simulink model "AQLRL"  (R2023b)
settings: Solver=FixedStepAuto  StartTime=0.0  StopTime=74.975  FixedStep=0.025  RelTol=1e-3
model workspace (MAT data in the model file):
  A : Simulink.Parameter (value not decoded)
  Aag : Simulink.Parameter (value not decoded)
  B : Simulink.Parameter (value not decoded)
  Bag : Simulink.Parameter (value not decoded)
  C : Simulink.Parameter (value not decoded)
  Cag : Simulink.Parameter (value not decoded)
  uang = [0 0 0 0 0 0 5.50670620214e-14 5.44009282066e-14 0 -3.99756362155e-05 -2.83106871279e-14 0 ... (9003 elements, 3x3001)]
  upos = [0 0 0 5.62466739851e-14 5.62327961973e-14 0 -2.39975660277e-05 4.94743135349e-14 0 -9.31686537426e-05 7.62168106405e-14 0 ... (9003 elements, 3x3001)]
values from neighbouring files (symbols this model uses):
  actions = [ ... (first row only)    [train_AQLRL.m]
  alpha = 0.5    [RL_iteration.m]    (also in RL_iteration2.m = 0.05; train_AQLRL.m = max(alpha * alpha_decay, alpha_min))
  epsilon = 0.4    [RL_iteration2.m]    (also in train_AQLRL.m = max(epsilon*epsilon_decay, epsilon_min))
  gamma = 0.9    [RL_iteration.m]    (also in RL_iteration2.m; train_AQLRL.m = 0.5)
  ref = [0 0 1.5 -3.29206127203e-06 0.00314263790126 1.5 -1.31682306379e-05 0.00628526200819 1.5 -2.96284647472e-05 0.00942785852649 1.5 ... (9000 elements, 3x3000)]    [circulartrajectory.mat]    (also in generate_circ_trajectory.m = [x;y;z]; generate_sprial_trajectory.m = [x;y;z]; generate_triangle_trajectory.m = [x;y;z]; spiralTrajectory.mat = [0 0 1.5 -2.96284647472e-05 0.00942785852649 1.50050016672 -)
  weights = evalin('base', 'weights')    [train_AQLRL.m]    (also in weights.mat = [0 0 0 0 0 0 0 0 0 0 0 0 ... (45 elements, 9x5)])
libraries: aerolibanimutils x1
(part 2 of 2)

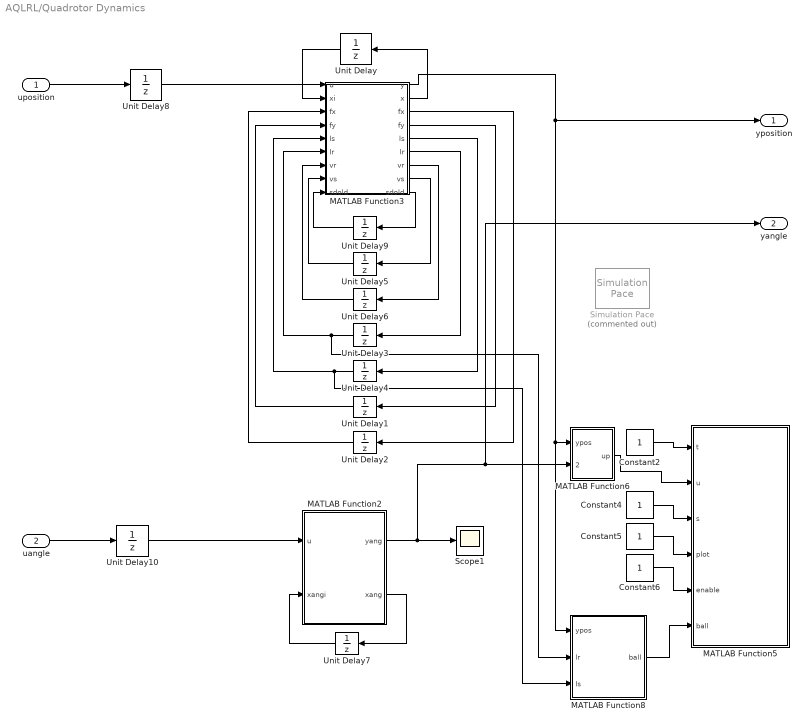
== system AQLRL/Quadrotor Dynamics ==
  uposition : Inport
  uangle : Inport  Port=2
  Constant{2,4..6} (4 alike) : Constant
  MATLAB Function2 : MATLAB Function  TreatAsAtomicUnit=on
  MATLAB Function3 : MATLAB Function  TreatAsAtomicUnit=on
  MATLAB Function5 : MATLAB Function  TreatAsAtomicUnit=on
  MATLAB Function6 : MATLAB Function  TreatAsAtomicUnit=on
  MATLAB Function8 : MATLAB Function  TreatAsAtomicUnit=on
  Scope1 : Scope
  Simulation Pace : aerolibanimutils/Simulation Pace  Commented=on  SimulationPace=1  SleepMode=Auto  OutputPaceError=off  SampleTime=-1
  Unit Delay : UnitDelay  InitialCondition=|  SampleTime=-1  HasFrameUpgradeWarning=on
      | [0
      | 0
      | 0
      | 0
      | 1.50000000000000
      | 0]
  Unit Delay{1..6,9} (7 alike) : UnitDelay  SampleTime=-1  HasFrameUpgradeWarning=on
  Unit Delay10 : UnitDelay  InitialCondition=|  SampleTime=-1  HasFrameUpgradeWarning=on
      | [0
      | 0
      | 0]
  Unit Delay7 : UnitDelay  InitialCondition=|  SampleTime=-1  HasFrameUpgradeWarning=on
      | [0
      | 0
      | 0
      | 0
      | 0
      | 0]
  Unit Delay8 : UnitDelay  InitialCondition=|  SampleTime=-1  HasFrameUpgradeWarning=on
      | [0
      | 0
      | 0]
  yposition : Outport
  yangle : Outport  Port=2
  wires:
  Unit Delay6/1 -> MATLAB Function3/7("vr ")
  MATLAB Function3/2(x) -> Unit Delay/1
  MATLAB Function3/5(ls) -> Unit Delay4/1
  MATLAB Function2/1(yang) -> Scope1/1, yangle/1, MATLAB Function6/2(yang)
  Constant4/1 -> MATLAB Function5/3(s)
  Constant2/1 -> MATLAB Function5/1(t)
  MATLAB Function3/4(fy) -> Unit Delay1/1
  Unit Delay/1 -> MATLAB Function3/2(xi)
  MATLAB Function3/9(sdold) -> Unit Delay9/1
  MATLAB Function8/1(ball) -> MATLAB Function5/6(ball)
  Unit Delay4/1 -> MATLAB Function8/3(ls), MATLAB Function3/5("ls ")
  Unit Delay2/1 -> MATLAB Function3/3("fx ")
  MATLAB Function2/2(xang) -> Unit Delay7/1
  MATLAB Function3/1(y) -> yposition/1, MATLAB Function8/1(ypos), MATLAB Function6/1(ypos)
  MATLAB Function3/6(lr) -> Unit Delay3/1
  Constant5/1 -> MATLAB Function5/4(plot)
  MATLAB Function3/8(vs) -> Unit Delay5/1
  Unit Delay3/1 -> MATLAB Function8/2(lr), MATLAB Function3/6("lr ")
  Unit Delay5/1 -> MATLAB Function3/8("vs ")
  Constant6/1 -> MATLAB Function5/5(enable)
  MATLAB Function6/1(up) -> MATLAB Function5/2(u)
  Unit Delay7/1 -> MATLAB Function2/2(xangi)
  MATLAB Function3/7(vr) -> Unit Delay6/1
  MATLAB Function3/3(fx) -> Unit Delay2/1
  Unit Delay9/1 -> MATLAB Function3/9("sdold ")
  Unit Delay1/1 -> MATLAB Function3/4("fy ")
  uposition/1 -> Unit Delay8/1
  uangle/1 -> Unit Delay10/1
  Unit Delay8/1 -> MATLAB Function3/1(u)
  Unit Delay10/1 -> MATLAB Function2/1(u)

== matlab function AQLRL/Quadrotor Dynamics/MATLAB Function5 ==
  data: t input; u input; s input; plot input; enable input; ball input
function qd_plot(t,u,s, plot, enable,ball)
    quad.nrotors =4;
    quad.d = 0.17;
    quad.r = 0.1;
    
    a1s = zeros(1, quad.nrotors);
    b1s = zeros(1, quad.nrotors);

    
    % vehicle dimensons
    d = quad.d; %Hub displacement from COG
    r = quad.r; %Rotor radius
    D = zeros(3,4);
    C = zeros(3,4);
    for i = 1:quad.nrotors
        theta = (i-1)/quad.nrotors*2*pi;
        %   Di      Rotor hub displacements (1x3)
        % first rotor is on the x-axis, clockwise order looking down from above
        D(:,i) = [ d*cos(theta); d*sin(theta); 0];
%         scal = s(1)/4;
        scal = 0.2/4;
        %Attitude center displacements
        C(:,i) = [ scal*cos(theta); scal*sin(theta); 0];
    end
    
    if enable == 1
        %draw ground
        figure(1);
        clf;
        if length(s) == 1
            axis([-0.5 1.5 -0.5 1.5 0 2]);
        else
%             axis([-s(1) s(1) -s(1) s(1) 0 s(2)])
            axis([-0.5 s(1) -0.5 s(1) 0 s(2)])
            s = 1.5;
        end
        hold on;
        
        % plot the ground boundaries and the big cross
        plot3([-0.5 -0.5],[-0.5 1],[0 0],'-b')
        plot3([-0.5 1.5],[-0.5 -0.5],[0 0],'-b')
        plot3([-0.5 1.5],[-0.5 1.5],[0 0],'-b')
        plot3([1.5 -0.5],[1.5 1.5],[0 0],'-b')
        plot3([1.5 1.5],[1.5 -0.5],[0 0],'-b')
        plot3([-0.5 1.5],[1.5 -0.5],[0 0],'-b')
        
        plot3([0 1], [0 0], [1.5 1.5],':r','LineWidth',0.2)
        plot3([1 1], [0 1], [1.5 1.5],':r','LineWidth',0.2)
        plot3([0 1], [1 1], [1.5 1.5],':r','LineWidth',0.2)
        plot3([0 0], [0 1], [1.5 1.5],':r','LineWidth',0.2)
        
        plot3([0 1], [0 0], [1 1],':r','LineWidth',0.2)
        plot3([1 1], [0 1], [1 1],':r','LineWidth',0.2)
        plot3([0 1], [1 1], [1 1],':r','LineWidth',0.2)
        plot3([0 0], [0 1], [1 1],':r','LineWidth',0.2)
        %READ STATE
        z = [u(1);u(2);u(3)];
        n = [u(4);u(5);u(6)];
        
        %PREPROCESS ROTATION MATRIX
        phi = n(1);    %Euler angles
        the = n(2);
        psi = n(3);
        
        R = [cos(the)*cos(phi) sin(psi)*sin(the)*cos(phi)-cos(psi)*sin(phi) cos(psi)*sin(the)*cos(phi)+sin(psi)*sin(phi);   %BBF > Inertial rotation matrix
            cos(the)*sin(phi) sin(psi)*sin(the)*sin(phi)+cos(psi)*cos(phi) cos(psi)*sin(the)*sin(phi)-sin(psi)*cos(phi);
            -sin(the)         sin(psi)*cos(the)                            cos(psi)*cos(the)];
        
        %Manual Construction
        %Q3 = [cos(psi) -sin(psi) 0;sin(psi) cos(psi) 0;0 0 1];   %Rotation mappings
        %Q2 = [cos(the) 0 sin(the);0 1 0;-sin(the) 0 cos(the)];
        %Q1 = [1 0 0;0 cos(phi) -sin(phi);0 sin(phi) cos(phi)];
        %R = Q3*Q2*Q1;    %Rotation matrix
        
        %CALCULATE FLYER TIP POSITONS USING COORDINATE FRAME ROTATION
        F = [1 0 0;0 -1 0;0 0 -1];
        
        %Draw flyer rotors
        t = [0:pi/8:2*pi];
        circle = zeros(3,17);
        for j = 1:length(t)
            circle(:,j) = [r*sin(t(j));r*cos(t(j));0];
        end
        hub = zeros(3,4);
        tippath = zeros(3,17,4);
        for i = 1:quad.nrotors
            hub(:,i) = F*(z + R*D(:,i)); %points in the inertial frame
            center = F*z;
            ball_pos = F*ball;
            plot3(center(1),center(2),center(3),'r.')
            plot3(ball_pos(1),ball_pos(2),ball_pos(3),'co')
            plot3([center(1) ball_pos(1)],[center(2) ball_pos(2)],[center(3) ball_pos(3)],'-b')
            
            q = 1; %Flapping angle scaling for output display - makes it easier to see what flapping is occurring
            Rr = [cos(q*a1s(i))  sin(q*b1s(i))*sin(q*a1s(i)) cos(q*b1s(i))*sin(q*a1s(i));   %Rotor > Plot frame
                0              cos(q*b1s(i))               -sin(q*b1s(i));
                -sin(q*a1s(i)) sin(q*b1s(i))*cos(q*a1s(i)) cos(q*b1s(i))*cos(q*a1s(i))];
            
            tippath(:,:,i) = F*R*Rr*circle;
            plot3([hub(1,i)+tippath(1,:,i)],[hub(2,i)+tippath(2,:,i)],[hub(3,i)+tippath(3,:,i)],'b-')
        end
        
        %Draw flyer
        hub0 = F*z;  % centre of vehicle
        for i = 1:quad.nrotors
            % line from hub to centre plot3([hub(1,N) hub(1,S)],[hub(2,N) hub(2,S)],[hub(3,N) hub(3,S)],'-b')
            plot3([hub(1,i) hub0(1)],[hub(2,i) hub0(2)],[hub(3,i) hub0(3)],'-b')
            
            % plot a circle at the hub itself
            plot3([hub(1,i)],[hub(2,i)],[hub(3,i)],'o')
        end
        
        % plot the vehicle's centroid on the ground plane
        plot3([z(1) 0],[-z(2) 0],[0 0],'--k')
        plot3([z(1)],[-z(2)],[0],'xk')
        plot3([z(1) z(1)],[-z(2) -s],[0 0],'r-.')

        % label the axes
        xlabel('x');
        ylabel('y');
        zlabel('z (height above ground)');
        view([-5 -2 5]);
    end;

== matlab function AQLRL/Quadrotor Dynamics/MATLAB Function6 ==
  data: up output; ypos input; yang input
function up= upp(ypos,yang)
up = [ypos(1) -ypos(2) -ypos(3) yang(1) yang(2) yang(3)];

== matlab function AQLRL/Quadrotor Dynamics/MATLAB Function8 ==
  data: ball output; ypos input; lr input; ls input
function ball= balll(ypos,lr,ls)
ball=[ypos(1)+lr(1) -(ypos(2)+ls(1)) 1-ypos(3)-sqrt(0.25-lr(1)^2-ls(1)^2)]';

== matlab function AQLRL/MATLAB Function1 ==
  data: features input; reward input; nextFeatures input; weights input size=[9,5]; newWeights output size=[9,5]; tdError output; alpha parameter; gamma parameter; actionIdx input size=[1,1]
function [newWeights, tdError] = Qupdate(features, reward, nextFeatures, weights, alpha, gamma, actionIdx)
% Approximate Q-learning weight update
% features      : current feature vector f(s,a)
% reward        : scalar reward at current step
% nextFeatures  : feature vector for next state-action
% weights       : current weight vector
%
% newWeights    : updated weights
% tdError       : temporal difference error (for debugging)

% Learning parameters
%alpha = 0.01; % learning rate (tune) 
%gamma = 0.95; % discount factor (tune) 
nextFeatures = nextFeatures(:); 
% Copy weights so we can modify
newWeights = weights; 

% Compute Q(s,a) for the chosen action 
Q_current = dot(weights(:, actionIdx), features); 

% Compute Q(s', a') for *best* next action
Q_next_vals = newWeights' * nextFeatures; % vector of Q-values for all actions
Q_next = max(Q_next_vals); 

% Temporal-difference error
tdError = reward + gamma * Q_next - Q_current; 

% Update only the chosen action column 
newWeights(:, actionIdx) = weights(:, actionIdx) + alpha * tdError * features;

== matlab function AQLRL/MATLAB Function ==
  data: state input size=[6,1]; R output; ref input size=[3,1]
function R  = RewardFcn(state, ref)
% RewardFcn - computes reward for quadrotor with suspended load
%
% Inputs:
%   state = [x, y, z, phi, theta, psi]   (from mux)
%   ref   = [x_ref, y_ref, z_ref]        (from squaretrajectory.mat at this timestep)
%
% Output:
%   R = scalar reward

% --- Extract state variables ---

x = state(1); 
y = state(2); 
z = state(3); 
phi = state(4); % roll
theta = state(5); % pitch
psi = state(6); % yaw


% Extract reference position 
x_ref = ref(1); 
y_ref = ref(2); 
z_ref = ref(3); 

% position error term (weighted)
R_pos = -(10*(x - x_ref)^2 + ...
           10*(y - y_ref)^2 + ...
           2*(z - z_ref) ^ 2); 

% angle stability term (penalize deviation from 0) 
R_angle = -((phi/10)^2 + (theta/10)^2 + (psi/10)^2); 

% Total reward
R = R_pos + R_angle;

== matlab function AQLRL/MATLAB Function2 ==
  data: state input size=[6,1]; features output size=[9,1]; ref input size=[3,1]
function features = FeatureBuilder(state, ref)
% state = [x, y, z, phi, theta, psi]
x = state(1); 
y = state(2); 
z = state(3); 
phi = state(4); 
theta = state(5); 
psi = state(6); 


% Compute errors against ref
x_err = x - ref(1); 
y_err = y - ref(2); 
z_err = z - ref(3); 

% build features 
features = [x_err; y_err; z_err; ...
            x_err^2; y_err^2; z_err^2; ...
            phi; theta; psi];

== matlab function AQLRL/MATLAB Function3 ==
  data: ref input; y output; t input
function y = fcn(ref, t)
T = floor(t/0.025)+1;
y = ref(:,T);

== matlab function AQLRL/MATLAB Function4 ==
  data: features input; action output size=[1,6]; weights input; epsilon input; actions input; idx output size=[1,1]
function [action,idx] = Qagent(features, weights, epsilon, actions)
% Qagent: epsilon-greedy action selection
%
% features: [nFeatures x 1]
% weights : [nFeatures x nActions]
% actions : [nActions x nControls] (defined in MATLAB script)
% epsilon : scalar exploration probability
%
% action : [1 x nControls] chosen control vector
features = features(:); 
numActions = size(actions, 1); % number of candidate actions

% Compute Q-values for each action
Q_values = zeros(1, numActions); 
for i = 1:numActions
    Q_values(i) = dot(weights(:,i), features); 

end 

% Epsilon-greedy choice
if rand < epsilon
    idx = randi(numActions); % random action 
else 
    [~, idx] = max(Q_values);  % greedy action 
end


% Output the chosen control vector
action = actions(idx,:); % row vector

== matlab function AQLRL/Quadrotor Dynamics/MATLAB Function2 ==
  data: yang output; xang output; u input; xangi input
function [yang,xang]= sysang(u,xangi)
Ts = 1/40;
g = 9.81;
A = [1,0.0250000000000000,0,0,0,0;0,1,0,0,0,0;0,0,1,0.0250000000000000,0,0;0,0,0,1,0,0;0,0,0,0,1,0.0250000000000000;0,0,0,0,0,1];
B = [0.0416666666666667,0,0;3.33333333333333,0,0;0,0.0416666666666667,0;0,3.33333333333333,0;0,0,0.0240384615384615;0,0,1.92307692307692];
C = [1,0,0,0,0,0;0,0,1,0,0,0;0,0,0,0,1,0];
D = zeros(3,3);
xang = zeros(6,1);
yang = zeros(3,1);
xang = A*xangi + B*u;
yang = C*xang + D*u;

== matlab function AQLRL/Quadrotor Dynamics/MATLAB Function3 ==
  data: y output; x output; u input; xi input; fx input; fy input; fx output; fy output; ls input; lr input; ls output; lr output; vr input; vs input; vr output; vs output; sdold input; sdold output
function [y,x, fx,fy,ls,lr,vr,vs,sdold]= syspos(u,xi,fx,fy,ls,lr,vr,vs,sdold)
Ts = 1/40;
g = 9.81;
A = [1 0.025 0 0 0 0;0 1 0 0 0 0;0 0 1 0.025 0 0;0 0 0 1 0 0;0 0 0 0 1 0.025;0 0 0 0 0 1];
B = [-0.003065625 0 0;-0.24525 0 0;0 0.003065625 0;0 0.24525 0;0 0 0.0003125;0 0 0.025];
C = [1 0 0 0 0 0;0 0 1 0 0 0;0 0 0 0 1 0];
D = zeros(3,3);
x = zeros(6,1);
y = zeros(3,1);
x = A*xi + B*u;
y = C*x + D*u;
x(2) = x(2) - fx;
x(4) = x(4) - fy;


xdold = x(2)-xi(2);
ydold = x(4)-xi(4);
zdold = x(6)-xi(6);

yita = sqrt(0.5^2-lr^2-ls^2);
vrold = vr;
vsold = vs;
vr = ( yita^4*xdold - lr*yita^3*zdold + lr*ls*yita^2*sdold +...
    (lr*0.5^2-lr*ls^2)*vr^2 +...
    (lr*0.5^2-lr^3)*vs^2 +...
    2*vr*vs*lr^2*ls + lr*g*yita^3 )/((ls^2-0.5^2)*yita^2);
lr = lr + vr*Ts;
rdold = vr-vrold;

vs = ( yita^4*ydold - ls*yita^3*zdold + lr*ls*yita^2*rdold +...
    (ls*0.5^2-ls*lr^2)*vs^2 +...
    (ls*0.5^2-ls^3)*vr^2 +...
    2*vr*vs*ls^2*lr + ls*g*yita^3 )/((lr^2-0.5^2)*yita^2);
ls = ls + vs*Ts;
% sdold = vs(1,i+1);
sdold = vs(1)-vsold(1);

fx = 0.3*(xdold+rdold);
fy = 0.3*(ydold+sdold);
